simulink model "data_acquisition_read_ds180b20"  (R2023b)
settings: Solver=FixedStepAuto  StartTime=0.0  StopTime=Inf  RelTol=1e-3  EnableMultiTasking=on
libraries: c2802xlib x4
settings Model: SimulationMode=external  ExtModeTrigDuration=8  Creator=Yamukelani  LastModifiedBy=yamzi
settings DataIOCC: LoggingToFile=on  LoggingFileName=C:\Users\yamzi\source_code\msc_research\rul_prediction\src\datasets\msc_rul_data.mat
settings OptimizationCC: DefaultUnderspecifiedDataType=single  EnhancedBackFolding=on  PassReuseOutputArgsAs=Individual arguments  MaxStackSize=768  OptimizeBlockOrder=speed  DifferentSizesBufferReuse=on  OptimizationCustomize=off  EfficientTunableParamExpr=on
settings DebuggingCC: ParameterTunabilityLossMsg=error
settings HardwareCC: ProdBitPerChar=16  ProdBitPerInt=16  ProdBitPerPointer=32  ProdBitPerSizeT=32  ProdBitPerPtrDiffT=32  ProdLargestAtomicInteger=Integer  ProdLargestAtomicFloat=None  ProdWordSize=16  ProdLongLongMode=on  ProdHWDeviceType=Texas Instruments->C2000
settings ModelReferenceCC: ModelReferenceNumInstancesAllowed=Single
settings SFSimCC: MATLABDynamicMemAlloc=off
settings RTWCC: Description=Embedded Coder  SystemTargetFile=ert.tlc  HardwareBoard=TI Piccolo F28027/F28027F LaunchPad  TemplateMakefile=ert_default_tmf  Toolchain=Texas Instruments Code Composer Studio (C2000)  CodeProfilingSaveOptions=MetricsOnly
settings CodeAppCC: ForceParamTrailComments=on  IgnoreCustomStorageClasses=off  OperatorAnnotations=on  SimulinkDataObjDesc=on  SFDataObjDesc=on  InsertBlockDesc=on
settings ERTTargetCC: CodeReplacementLibrary=TI C28x  ExtMode=on  ExtModeTransport=4  ExtModeStaticAlloc=on  ExtModeAutomaticAllocSize=off  ExtModeStaticAllocSize=500  ExtModeMexFile=ext_xcp  ExtModeMexArgs=1 5 3750000  ExtModeIntrfLevel=Level2 - Open

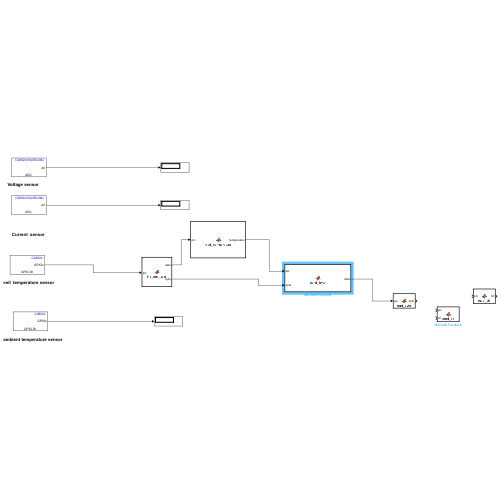
[thumbnail: Simulink's stored preview of the top-level diagram]
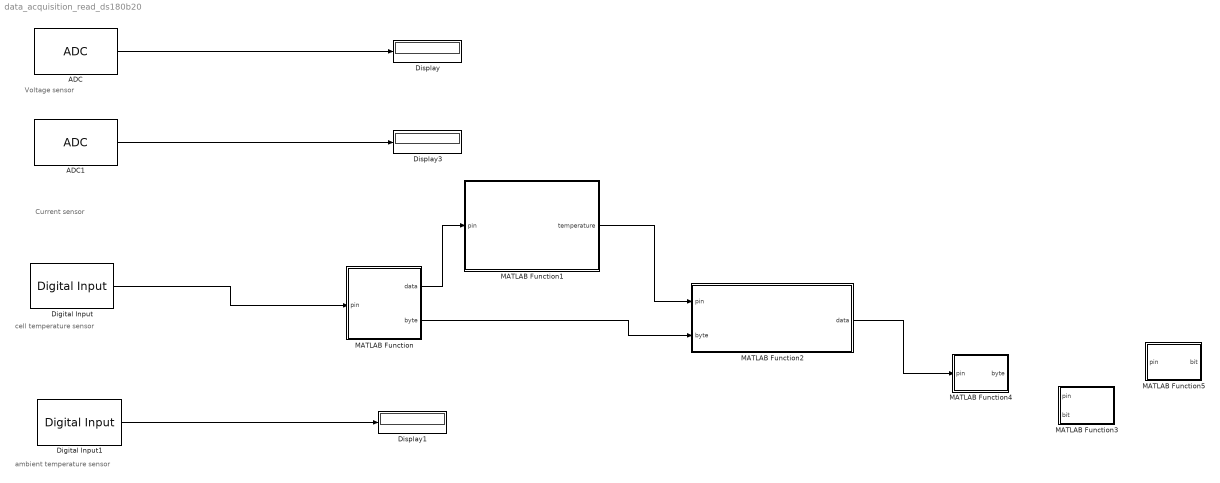
== system data_acquisition_read_ds180b20 ==
  note: ambient temperature sensor
  note: cell temperature sensor
  note: Current sensor
  note: Voltage sensor
  ADC : c2802xlib/ADC  blkParamProc=C2000  ADCModule=1  samplingMode=Single sample mode  ADCResolution=12-bit (Single-ended input)  useSOC1=SOC0  useSOC2=SOC0_SOC1  SOCAcquisitionWindow=7  SOCTriggerSource=CPU0_TINT0n  SOCInterruptTrigger=No ADCINT  Ts=0.005  dType=uint16  postInterrupt=off  interruptSel=ADCINT1  ADCINTContinuous=on  endma=off  chdma=1  conv1=ADCINA0  conv2=ADCINA0 and ADCINB0  conv1_Type4=ADCIN0  conv2_Type4=ADCIN0 and ADCIN1
  ADC1 : c2802xlib/ADC  blkParamProc=C2000  ADCModule=1  samplingMode=Single sample mode  ADCResolution=12-bit (Single-ended input)  useSOC1=SOC1  useSOC2=SOC0_SOC1  SOCAcquisitionWindow=7  SOCTriggerSource=CPU0_TINT0n  SOCInterruptTrigger=No ADCINT  Ts=0.005  dType=uint16  postInterrupt=off  interruptSel=ADCINT1  ADCINTContinuous=on  endma=off  chdma=1  conv1=ADCINA3  conv2=ADCINA0 and ADCINB0  conv1_Type4=ADCIN0  conv2_Type4=ADCIN0 and ADCIN1
  Digital Input : c2802xlib/Digital Input  GPIO_Number=GPIO0~GPIO7  GPIO_Bit0=on  GPIO_Bit1=off  GPIO_Bit2=off  GPIO_Bit3=off  GPIO_Bit4=off  GPIO_Bit5=off  GPIO_Bit6=off  GPIO_Bit7=off  sampleTime=0.5  dataType=double  GPIO_Bit0_Qualification=Sync to SYSCLKOUT  GPIO_Bit1_Qualification=Sync to SYSCLKOUT  GPIO_Bit2_Qualification=Sync to SYSCLKOUT  GPIO_Bit3_Qualification=Sync to SYSCLKOUT  GPIO_Bit4_Qualification=Sync to SYSCLKOUT  GPIO_Bit5_Qualification=Sync to SYSCLKOUT  GPIO_Bit6_Qualification=Sync to SYSCLKOUT  GPIO_Bit7_Qualification=Sync to SYSCLKOUT  Qualification_Period=-1
  Digital Input1 : c2802xlib/Digital Input  Tag=ambient_temperature  GPIO_Number=GPIO0~GPIO7  GPIO_Bit0=off  GPIO_Bit1=on  GPIO_Bit2=off  GPIO_Bit3=off  GPIO_Bit4=off  GPIO_Bit5=off  GPIO_Bit6=off  GPIO_Bit7=off  sampleTime=0.5  dataType=auto  GPIO_Bit0_Qualification=Sync to SYSCLKOUT  GPIO_Bit1_Qualification=Sync to SYSCLKOUT  GPIO_Bit2_Qualification=Sync to SYSCLKOUT  GPIO_Bit3_Qualification=Sync to SYSCLKOUT  GPIO_Bit4_Qualification=Sync to SYSCLKOUT  GPIO_Bit5_Qualification=Sync to SYSCLKOUT  GPIO_Bit6_Qualification=Sync to SYSCLKOUT  GPIO_Bit7_Qualification=Sync to SYSCLKOUT  Qualification_Period=-1
  Display : Display
  Display1 : Display
  Display3 : Display
  MATLAB Function : MATLAB Function  TreatAsAtomicUnit=on
  MATLAB Function1 : MATLAB Function  TreatAsAtomicUnit=on
  MATLAB Function2 : MATLAB Function  TreatAsAtomicUnit=on
  MATLAB Function3 : MATLAB Function  TreatAsAtomicUnit=on
  MATLAB Function4 : MATLAB Function  TreatAsAtomicUnit=on
  MATLAB Function5 : MATLAB Function  TreatAsAtomicUnit=on
  wires:
  ADC/1 -> Display/1
  ADC1/1 -> Display3/1
  Digital Input/1 -> MATLAB Function/1(pin)
  Digital Input1/1 -> Display1/1
  MATLAB Function/1(data) -> MATLAB Function1/1(pin)
  MATLAB Function1/1(temperature) -> MATLAB Function2/1(pin)
  MATLAB Function/2(byte) -> MATLAB Function2/2(byte)
  MATLAB Function2/1(data) -> MATLAB Function4/1(pin)

== matlab function data_acquisition_read_ds180b20/MATLAB Function ==
  data: pin input; data output; byte output
function [data,byte] = init_one_wire(pin)
    % Initialize the DS18B20 sensor
    coder.cinclude('DSP28x_Project.h');
    coder.cinclude('DSP2833x_Gpio.h');
    
    % Drive the pin low
    coder.ceval('GpioDataRegs.GPACLEAR.bit.GPIO' + num2str(pin) + ' = 1;');
    pause(0.00048); % 480us delay
    
    % Release the pin
    coder.ceval('GpioDataRegs.GPASET.bit.GPIO' + num2str(pin) + ' = 1;');
    pause(0.00007); % 70us delay
end

== matlab function data_acquisition_read_ds180b20/MATLAB Function2 ==
  data: pin input; byte input; data output
function data = send_byte(pin, byte)
    for i = 0:7
        send_bit(pin, bitand(byte, 1));
        byte = bitshift(byte, -1);
    end
end

== matlab function data_acquisition_read_ds180b20/MATLAB Function3 ==
  data: pin input; bit input
function send_bit(pin, bit)
    coder.cinclude('DSP28x_Project.h');
    coder.cinclude('DSP2833x_Gpio.h');
    
    if bit == 1
        % Write 1
        coder.ceval('GpioDataRegs.GPACLEAR.bit.GPIO' + num2str(pin) + ' = 1;');
        pause(0.000001); % 1us delay
        coder.ceval('GpioDataRegs.GPASET.bit.GPIO' + num2str(pin) + ' = 1;');
        pause(0.000060); % 60us delay
    else
        % Write 0
        coder.ceval('GpioDataRegs.GPACLEAR.bit.GPIO' + num2str(pin) + ' = 1;');
        pause(0.000060); % 60us delay
        coder.ceval('GpioDataRegs.GPASET.bit.GPIO' + num2str(pin) + ' = 1;');
        pause(0.000001); % 1us delay
    end
end

== matlab function data_acquisition_read_ds180b20/MATLAB Function4 ==
  data: pin input; byte output
function byte = read_byte(pin)
    byte = 0;
    for i = 0:7
        byte = bitor(byte, bitshift(read_bit(pin), i));
    end
end

== matlab function data_acquisition_read_ds180b20/MATLAB Function5 ==
  data: pin input; bit output
function bit = read_bit(pin)
    coder.cinclude('DSP28x_Project.h');
    coder.cinclude('DSP2833x_Gpio.h');
    
    % Drive the pin low
    coder.ceval('GpioDataRegs.GPACLEAR.bit.GPIO' + num2str(pin) + ' = 1;');
    pause(0.000001); % 1us delay
    
    % Release the pin
    coder.ceval('GpioDataRegs.GPASET.bit.GPIO' + num2str(pin) + ' = 1;');
    pause(0.000015); % 15us delay
    
    % Read the pin state
    bit = coder.ceval('GpioDataRegs.GPADAT.bit.GPIO' + num2str(pin) + ';');
    pause(0.000045); % 45us delay
end

== matlab function data_acquisition_read_ds180b20/MATLAB Function1 ==
  data: pin input; temperature output
function temperature = read_temperature(pin)
    % Read temperature from DS18B20
    init_one_wire(pin);
    
    % Send the Skip ROM command (0xCC)
    send_byte(pin, hex2dec('CC'));
    
    % Send the Convert T command (0x44)
    send_byte(pin, hex2dec('44'));
    
    pause(0.75); % Wait for temperature conversion (750ms)
    
    init_one_wire(pin);
    
    % Send the Skip ROM command (0xCC)
    send_byte(pin, hex2dec('CC'));
    
    % Send the Read Scratchpad command (0xBE)
    send_byte(pin, hex2dec('BE'));
    
    % Read 2 bytes (temperature data)
    lsb = read_byte(pin);
    msb = read_byte(pin);
    
    % Calculate the temperature
    temperature = ((msb << 8) | lsb) * 0.0625;
end
